simulink model "hcu_main_ADASwEPS"  (Simulink 8.2)
settings: Solver=FixedStepDiscrete  StartTime=0.0  StopTime=inf  FixedStep=0.001  RelTol=1e-3
PostLoadFcn:
  | , if any(exist('dsrtsu_mdlpostloadfcn', 'file') == [2, 3, 6]), try dsrtsu_mdlpostloadfcn('Execute', bdroot); catch fprintf('Error in PostLoadFcn (dsrtsu_mdlpostloadfcn) for model "%s":\n %s\n', bdroot, lasterr); end, end,
values from neighbouring files (symbols this model uses):
  C_TASK_1MS_S = (	C_TICK_TIME_S       )    [hcu_local_hdr.m]    (also in temp_ovrd_values.m = double(	0.001                  ))
  C_TASK_5MS_S = (	C_TICK_TIME_S      	)    [hcu_local_hdr.m]
  ENUM_ADASLFCSTATUS_OFF = uint8(  0  )    [hcu_local_hdr.m]
  ENUM_ADASLFCSTATUS_STANDBY = uint8(  1  )    [hcu_local_hdr.m]
  ENUM_ADASLKASTATUS_ACTIVE = uint8(  2  )    [hcu_local_hdr.m]
  ENUM_ADASLKASTATUS_OFF = uint8(  0  )    [hcu_local_hdr.m]
  ENUM_ADASLKASTATUS_STANDBY = uint8(  1  )    [hcu_local_hdr.m]
  ENUM_EPSMODEREQ_ANGLE = uint8(  1  )    [hcu_local_hdr.m]
  ENUM_EPSMODEREQ_INTERNAL = uint8(  0  )    [hcu_local_hdr.m]
  ENUM_EPSMODEREQ_TORQUE = uint8(  2  )    [hcu_local_hdr.m]
  ENUM_GEARPOSN_1ST = uint8(  1  )    [hcu_local_hdr.m]
  ENUM_GEARPOSN_2ND = uint8(  2  )    [hcu_local_hdr.m]
  ENUM_GEARPOSN_3RD = uint8(  3  )    [hcu_local_hdr.m]
  ENUM_GEARPOSN_4TH = uint8(  4  )    [hcu_local_hdr.m]
  ENUM_GEARPOSN_5TH = uint8(  5  )    [hcu_local_hdr.m]
  ENUM_GEARPOSN_6TH = uint8(  6  )    [hcu_local_hdr.m]
  ENUM_GEARPOSN_PN = uint8(  0  )    [hcu_local_hdr.m]
  ENUM_GEARPOSN_R = uint8(  7  )    [hcu_local_hdr.m]
  FALSE = boolean( 0 )    [hcu_local_hdr.m]
  TRUE = boolean( 1 )    [hcu_local_hdr.m]
undefined symbols (not defined in the file or in its folder): AACC_DistCtrlIMult_X_mps2, AACC_DistCtrlPMult_X_mps2, AACC_GearActual_enum, AACC_SpdCtrlIMult_X_mps2, AACC_SpdCtrlPMult_X_mps2, AACC_VehSpd_kph, AISP_EPSCurrent_pct, AISP_TqASensorDelta_pct, AISP_TqBSensorDelta_pct, ENUM_ACCSTATUS_ACTIVE, ENUM_ACCSTATUS_OFF, ENUM_ACCSTATUS_STANDBY, ENUM_ADASLFCSTATUS_ACTIVE, ENUM_ADASLFCSTATUS_TRANSITION, ENUM_LFCCCONTSTATUS_ACTIVE, ENUM_LFCCCONTSTATUS_NOTAVAIL_TEMP, ENUM_LFCCCONTSTATUS_OFF, ENUM_LFCCCONTSTATUS_READY, ENUM_LFCCCONTSTATUS_TRANSITION, ENUM_LKACCONTSTATUS_ACTIVE, ENUM_LKACCONTSTATUS_NOTAVAIL_TEMP, ENUM_LKACCONTSTATUS_OFF, ENUM_LKACCONTSTATUS_READY, KACC_AcclReqMax_g, KACC_AcclReqMin_g, KACC_ACCSetTimeGapDef1_s, KACC_ACCSetTimeGapDef2_s, KACC_ACCSetTimeGapDef3_s, KACC_ACCSetTimeGapDef4_s, KACC_ACCSetTimeGapDef5_s, KACC_AirDensity_kgpm3, KACC_AirDragCoef_rat, KACC_CommandsOn_flg, KACC_CruzSpdChgTimeThres_s, KACC_DecReqSwOffThres_Nm, KACC_DecReqSwOnThres_Nm, KACC_DistCtrlAdjTime_s, KACC_DistCtrlCalRate_s, KACC_DistCtrlIC_mps2, KACC_DistCtrlIGain_rat, KACC_DistCtrlIMax_mps2, KACC_DistCtrlIMin_mps2, KACC_DistCtrlIRest_flg, KACC_DistCtrlKGain_rat, KACC_DistCtrlPause_flg, KACC_DistCtrlPGain_rat, KACC_FinalDriveEff_pct, KACC_FinalDriveRatio_rat, KACC_FrontalArea_m2, KACC_GearBoxEff_pct, KACC_LongPushSpdChg_kph, KACC_MaxAccSetSpd_kph, KACC_MinAccSetSpd_kph, KACC_SetAllowSpdLim_kph, KACC_SpdCtrlAdjTime_s, KACC_SpdCtrlCalRate_s, KACC_SpdCtrlIC_mps2, KACC_SpdCtrlIGain_rat, KACC_SpdCtrlIMax_mps2, KACC_SpdCtrlIMin_mps2 ... (+26)
libraries: simulink x54, adas_lib x6, rti1401lib_dio_type3 x4, rtimmsu_dsrtlib x3, hcu_lib x2, aeb x1, ddm x1, dfr x1, dgi x1, dhp x1, dinr x1, dip x1
(part 4 of 9)

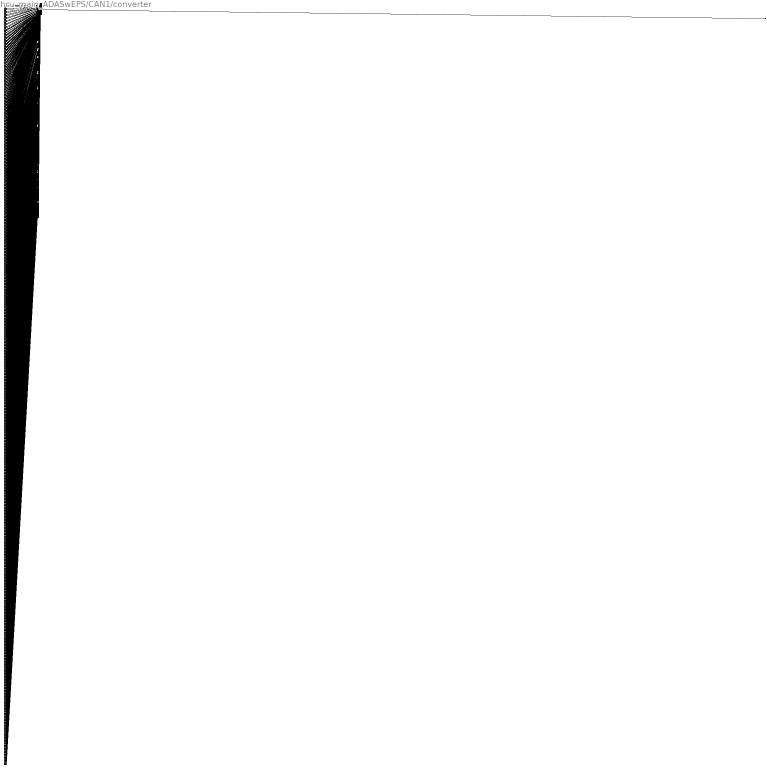
== system hcu_main_ADASwEPS/CAN1/converter ==
  in_1 : Inport
  in_2 : Inport  Port=2
  in_3 : Inport  Port=3
  in_4 : Inport  Port=4
  in_5 : Inport  Port=5
  in_6 : Inport  Port=6
  in_7 : Inport  Port=7
  in_8 : Inport  Port=8
  in_9 : Inport  Port=9
  in_10 : Inport  Port=10
  in_11 : Inport  Port=11
  in_12 : Inport  Port=12
  in_13 : Inport  Port=13
  in_14 : Inport  Port=14
  in_15 : Inport  Port=15
  in_16 : Inport  Port=16
  in_17 : Inport  Port=17
  in_18 : Inport  Port=18
  in_19 : Inport  Port=19
  in_20 : Inport  Port=20
  in_21 : Inport  Port=21
  in_22 : Inport  Port=22
  in_23 : Inport  Port=23
  in_24 : Inport  Port=24
  in_25 : Inport  Port=25
  in_26 : Inport  Port=26
  in_27 : Inport  Port=27
  in_28 : Inport  Port=28
  in_29 : Inport  Port=29
  in_30 : Inport  Port=30
  in_31 : Inport  Port=31
  in_32 : Inport  Port=32
  in_33 : Inport  Port=33
  in_34 : Inport  Port=34
  in_35 : Inport  Port=35
  in_36 : Inport  Port=36
  in_37 : Inport  Port=37
  in_38 : Inport  Port=38
  in_39 : Inport  Port=39
  in_40 : Inport  Port=40
  in_41 : Inport  Port=41
  in_42 : Inport  Port=42
  in_43 : Inport  Port=43
  in_44 : Inport  Port=44
  in_45 : Inport  Port=45
  in_46 : Inport  Port=46
  in_47 : Inport  Port=47
  in_48 : Inport  Port=48
  in_49 : Inport  Port=49
  in_50 : Inport  Port=50
  in_51 : Inport  Port=51
  in_52 : Inport  Port=52
  in_53 : Inport  Port=53
  in_54 : Inport  Port=54
  in_55 : Inport  Port=55
  in_56 : Inport  Port=56
  in_57 : Inport  Port=57
  in_58 : Inport  Port=58
  in_59 : Inport  Port=59
  in_60 : Inport  Port=60
  in_61 : Inport  Port=61
  in_62 : Inport  Port=62
  in_63 : Inport  Port=63
  in_64 : Inport  Port=64
  in_65 : Inport  Port=65
  in_66 : Inport  Port=66
  in_67 : Inport  Port=67
  in_68 : Inport  Port=68
  in_69 : Inport  Port=69
  in_70 : Inport  Port=70
  in_71 : Inport  Port=71
  in_72 : Inport  Port=72
  in_73 : Inport  Port=73
  in_74 : Inport  Port=74
  in_75 : Inport  Port=75
  in_76 : Inport  Port=76
  in_77 : Inport  Port=77
  in_78 : Inport  Port=78
  in_79 : Inport  Port=79
  in_80 : Inport  Port=80
  in_81 : Inport  Port=81
  in_82 : Inport  Port=82
  in_83 : Inport  Port=83
  in_84 : Inport  Port=84
  in_85 : Inport  Port=85
  in_86 : Inport  Port=86
  in_87 : Inport  Port=87
  in_88 : Inport  Port=88
  in_89 : Inport  Port=89
  in_90 : Inport  Port=90
  in_91 : Inport  Port=91
  in_92 : Inport  Port=92
  in_93 : Inport  Port=93
  in_94 : Inport  Port=94
  in_95 : Inport  Port=95
  in_96 : Inport  Port=96
  in_97 : Inport  Port=97
  in_98 : Inport  Port=98
  in_99 : Inport  Port=99
  in_100 : Inport  Port=100
  in_101 : Inport  Port=101
  in_102 : Inport  Port=102
  in_103 : Inport  Port=103
  in_104 : Inport  Port=104
  in_105 : Inport  Port=105
  in_106 : Inport  Port=106
  in_107 : Inport  Port=107
  in_108 : Inport  Port=108
  in_109 : Inport  Port=109
  in_110 : Inport  Port=110
  in_111 : Inport  Port=111
  in_112 : Inport  Port=112
  in_113 : Inport  Port=113
  in_114 : Inport  Port=114
  in_115 : Inport  Port=115
  in_116 : Inport  Port=116
  in_117 : Inport  Port=117
  in_118 : Inport  Port=118
  in_119 : Inport  Port=119
  in_120 : Inport  Port=120
  in_121 : Inport  Port=121
  in_122 : Inport  Port=122
  in_123 : Inport  Port=123
  in_124 : Inport  Port=124
  in_125 : Inport  Port=125
  in_126 : Inport  Port=126
  in_127 : Inport  Port=127
  in_128 : Inport  Port=128
  in_129 : Inport  Port=129
  in_130 : Inport  Port=130
  in_131 : Inport  Port=131
  in_132 : Inport  Port=132
  in_133 : Inport  Port=133
  in_134 : Inport  Port=134
  in_135 : Inport  Port=135
  in_136 : Inport  Port=136
  in_137 : Inport  Port=137
  in_138 : Inport  Port=138
  in_139 : Inport  Port=139
  in_140 : Inport  Port=140
  in_141 : Inport  Port=141
  in_142 : Inport  Port=142
  in_143 : Inport  Port=143
  in_144 : Inport  Port=144
  in_145 : Inport  Port=145
  in_146 : Inport  Port=146
  in_147 : Inport  Port=147
  in_148 : Inport  Port=148
  in_149 : Inport  Port=149
  in_150 : Inport  Port=150
  in_151 : Inport  Port=151
  in_152 : Inport  Port=152
  in_153 : Inport  Port=153
  in_154 : Inport  Port=154
  in_155 : Inport  Port=155
  in_156 : Inport  Port=156
  in_157 : Inport  Port=157
  in_158 : Inport  Port=158
  in_159 : Inport  Port=159
  in_160 : Inport  Port=160
  in_161 : Inport  Port=161
  in_162 : Inport  Port=162
  in_163 : Inport  Port=163
  in_164 : Inport  Port=164
  in_165 : Inport  Port=165
  in_166 : Inport  Port=166
  in_167 : Inport  Port=167
  in_168 : Inport  Port=168
  in_169 : Inport  Port=169
  in_170 : Inport  Port=170
  in_171 : Inport  Port=171
  in_172 : Inport  Port=172
  in_173 : Inport  Port=173
  in_174 : Inport  Port=174
  in_175 : Inport  Port=175
  in_176 : Inport  Port=176
  in_177 : Inport  Port=177
  in_178 : Inport  Port=178
  in_179 : Inport  Port=179
  in_180 : Inport  Port=180
  in_181 : Inport  Port=181
  in_182 : Inport  Port=182
  in_183 : Inport  Port=183
  in_184 : Inport  Port=184
  in_185 : Inport  Port=185
  in_186 : Inport  Port=186
  in_187 : Inport  Port=187
  in_188 : Inport  Port=188
  in_189 : Inport  Port=189
  in_190 : Inport  Port=190
  in_191 : Inport  Port=191
  in_192 : Inport  Port=192
  in_193 : Inport  Port=193
  in_194 : Inport  Port=194
  in_195 : Inport  Port=195
  in_196 : Inport  Port=196
  in_197 : Inport  Port=197
  in_198 : Inport  Port=198
  in_199 : Inport  Port=199
  in_200 : Inport  Port=200
  in_201 : Inport  Port=201
  in_202 : Inport  Port=202
  in_203 : Inport  Port=203
  in_204 : Inport  Port=204
  in_205 : Inport  Port=205
  in_206 : Inport  Port=206
  in_207 : Inport  Port=207
  in_208 : Inport  Port=208
  in_209 : Inport  Port=209
  in_210 : Inport  Port=210
  in_211 : Inport  Port=211
  in_212 : Inport  Port=212
  in_213 : Inport  Port=213
  in_214 : Inport  Port=214
  in_215 : Inport  Port=215
  in_216 : Inport  Port=216
  in_217 : Inport  Port=217
  in_218 : Inport  Port=218
  in_219 : Inport  Port=219
  in_220 : Inport  Port=220
  in_221 : Inport  Port=221
  in_222 : Inport  Port=222
  in_223 : Inport  Port=223
  in_224 : Inport  Port=224
  in_225 : Inport  Port=225
  in_226 : Inport  Port=226
  in_227 : Inport  Port=227
  in_228 : Inport  Port=228
  in_229 : Inport  Port=229
  in_230 : Inport  Port=230
  in_231 : Inport  Port=231
  in_232 : Inport  Port=232
  in_233 : Inport  Port=233
  in_234 : Inport  Port=234
  in_235 : Inport  Port=235
  in_236 : Inport  Port=236
  in_237 : Inport  Port=237
  in_238 : Inport  Port=238
  in_239 : Inport  Port=239
  in_240 : Inport  Port=240
  in_241 : Inport  Port=241
  in_242 : Inport  Port=242
  in_243 : Inport  Port=243
  in_244 : Inport  Port=244
  in_245 : Inport  Port=245
  in_246 : Inport  Port=246
  in_247 : Inport  Port=247
  in_248 : Inport  Port=248
  in_249 : Inport  Port=249
  in_250 : Inport  Port=250
  in_251 : Inport  Port=251
  in_252 : Inport  Port=252
  in_253 : Inport  Port=253
  in_254 : Inport  Port=254
  in_255 : Inport  Port=255
  in_256 : Inport  Port=256
  in_257 : Inport  Port=257
  in_258 : Inport  Port=258
  in_259 : Inport  Port=259
  in_260 : Inport  Port=260
  in_261 : Inport  Port=261
  in_262 : Inport  Port=262
  in_263 : Inport  Port=263
  in_264 : Inport  Port=264
  in_265 : Inport  Port=265
  in_266 : Inport  Port=266
  in_267 : Inport  Port=267
  in_268 : Inport  Port=268
  in_269 : Inport  Port=269
  in_270 : Inport  Port=270
  in_271 : Inport  Port=271
  in_272 : Inport  Port=272
  in_273 : Inport  Port=273
  in_274 : Inport  Port=274
  in_275 : Inport  Port=275
  in_276 : Inport  Port=276
  in_277 : Inport  Port=277
  in_278 : Inport  Port=278
  in_279 : Inport  Port=279
  in_280 : Inport  Port=280
  in_281 : Inport  Port=281
  in_282 : Inport  Port=282
  in_283 : Inport  Port=283
  in_284 : Inport  Port=284
  in_285 : Inport  Port=285
  in_286 : Inport  Port=286
  in_287 : Inport  Port=287
  in_288 : Inport  Port=288
  in_289 : Inport  Port=289
  in_290 : Inport  Port=290
  in_291 : Inport  Port=291
  in_292 : Inport  Port=292
  in_293 : Inport  Port=293
  in_294 : Inport  Port=294
  in_295 : Inport  Port=295
  in_296 : Inport  Port=296
  in_297 : Inport  Port=297
  in_298 : Inport  Port=298
  in_299 : Inport  Port=299
  in_300 : Inport  Port=300
  in_301 : Inport  Port=301
  in_302 : Inport  Port=302
  in_303 : Inport  Port=303
  in_304 : Inport  Port=304
  in_305 : Inport  Port=305
  in_306 : Inport  Port=306
  in_307 : Inport  Port=307
  in_308 : Inport  Port=308
  in_309 : Inport  Port=309
  in_310 : Inport  Port=310
  in_311 : Inport  Port=311
  in_312 : Inport  Port=312
  in_313 : Inport  Port=313
  in_314 : Inport  Port=314
  in_315 : Inport  Port=315
  in_316 : Inport  Port=316
  in_317 : Inport  Port=317
  in_318 : Inport  Port=318
  in_319 : Inport  Port=319
  in_320 : Inport  Port=320
  in_321 : Inport  Port=321
  in_322 : Inport  Port=322
  in_323 : Inport  Port=323
  in_324 : Inport  Port=324
  in_325 : Inport  Port=325
  in_326 : Inport  Port=326
  in_327 : Inport  Port=327
  in_328 : Inport  Port=328
  in_329 : Inport  Port=329
  in_330 : Inport  Port=330
  in_331 : Inport  Port=331
  in_332 : Inport  Port=332
  in_333 : Inport  Port=333
  in_334 : Inport  Port=334
  in_335 : Inport  Port=335
  in_336 : Inport  Port=336
  in_337 : Inport  Port=337
  in_338 : Inport  Port=338
  in_339 : Inport  Port=339
  in_340 : Inport  Port=340
  in_341 : Inport  Port=341
  in_342 : Inport  Port=342
  in_343 : Inport  Port=343
  in_344 : Inport  Port=344
  in_345 : Inport  Port=345
  in_346 : Inport  Port=346
  in_347 : Inport  Port=347
  in_348 : Inport  Port=348
  in_349 : Inport  Port=349
  in_350 : Inport  Port=350
  in_351 : Inport  Port=351
  in_352 : Inport  Port=352
  in_353 : Inport  Port=353
  in_354 : Inport  Port=354
  in_355 : Inport  Port=355
  in_356 : Inport  Port=356
  in_357 : Inport  Port=357
  in_358 : Inport  Port=358
  in_359 : Inport  Port=359
  in_360 : Inport  Port=360
  in_361 : Inport  Port=361
  in_362 : Inport  Port=362
  in_363 : Inport  Port=363
  in_364 : Inport  Port=364
  in_365 : Inport  Port=365
  in_366 : Inport  Port=366
  in_367 : Inport  Port=367
  in_368 : Inport  Port=368
  in_369 : Inport  Port=369
  in_370 : Inport  Port=370
  in_371 : Inport  Port=371
  in_372 : Inport  Port=372
  in_373 : Inport  Port=373
  in_374 : Inport  Port=374
  in_375 : Inport  Port=375
  in_376 : Inport  Port=376
  in_377 : Inport  Port=377
  in_378 : Inport  Port=378
  in_379 : Inport  Port=379
  in_380 : Inport  Port=380
  in_381 : Inport  Port=381
  in_382 : Inport  Port=382
  in_383 : Inport  Port=383
  in_384 : Inport  Port=384
  in_385 : Inport  Port=385
  in_386 : Inport  Port=386
  in_387 : Inport  Port=387
  in_388 : Inport  Port=388
  in_389 : Inport  Port=389
  in_390 : Inport  Port=390
  in_391 : Inport  Port=391
  in_392 : Inport  Port=392
  in_393 : Inport  Port=393
  in_394 : Inport  Port=394
  in_395 : Inport  Port=395
  in_396 : Inport  Port=396
  in_397 : Inport  Port=397
  in_398 : Inport  Port=398
  in_399 : Inport  Port=399
  in_400 : Inport  Port=400
  in_401 : Inport  Port=401
  in_402 : Inport  Port=402
  in_403 : Inport  Port=403
  in_404 : Inport  Port=404
  in_405 : Inport  Port=405
  in_406 : Inport  Port=406
  in_407 : Inport  Port=407
  in_408 : Inport  Port=408
  in_409 : Inport  Port=409
  in_410 : Inport  Port=410
  in_411 : Inport  Port=411
  in_412 : Inport  Port=412
  in_413 : Inport  Port=413
  in_414 : Inport  Port=414
  in_415 : Inport  Port=415
  in_416 : Inport  Port=416
  in_417 : Inport  Port=417
  in_418 : Inport  Port=418
  in_419 : Inport  Port=419
  in_420 : Inport  Port=420
  in_421 : Inport  Port=421
  in_422 : Inport  Port=422
  in_423 : Inport  Port=423
  in_424 : Inport  Port=424
  in_425 : Inport  Port=425
  in_426 : Inport  Port=426
  in_427 : Inport  Port=427
  in_428 : Inport  Port=428
  in_429 : Inport  Port=429
  in_430 : Inport  Port=430
  in_431 : Inport  Port=431
  in_432 : Inport  Port=432
  in_433 : Inport  Port=433
  in_434 : Inport  Port=434
  in_435 : Inport  Port=435
  in_436 : Inport  Port=436
  in_437 : Inport  Port=437
  in_438 : Inport  Port=438
  in_439 : Inport  Port=439
  in_440 : Inport  Port=440
  in_441 : Inport  Port=441
  in_442 : Inport  Port=442
  in_443 : Inport  Port=443
  in_444 : Inport  Port=444
  in_445 : Inport  Port=445
  in_446 : Inport  Port=446
  in_447 : Inport  Port=447
  in_448 : Inport  Port=448
  in_449 : Inport  Port=449
  in_450 : Inport  Port=450
  in_451 : Inport  Port=451
  in_452 : Inport  Port=452
  in_453 : Inport  Port=453
  in_454 : Inport  Port=454
  in_455 : Inport  Port=455
  in_456 : Inport  Port=456
  in_457 : Inport  Port=457
  in_458 : Inport  Port=458
  in_459 : Inport  Port=459
  in_460 : Inport  Port=460
  in_461 : Inport  Port=461
  in_462 : Inport  Port=462
  in_463 : Inport  Port=463
  in_464 : Inport  Port=464
  in_465 : Inport  Port=465
  in_466 : Inport  Port=466
  in_467 : Inport  Port=467
  in_468 : Inport  Port=468
  in_469 : Inport  Port=469
  in_470 : Inport  Port=470
  in_471 : Inport  Port=471
  in_472 : Inport  Port=472
  in_473 : Inport  Port=473
  in_474 : Inport  Port=474
  in_475 : Inport  Port=475
  in_476 : Inport  Port=476
  in_477 : Inport  Port=477
  in_478 : Inport  Port=478
  in_479 : Inport  Port=479
  in_480 : Inport  Port=480
  in_481 : Inport  Port=481
  in_482 : Inport  Port=482
  in_483 : Inport  Port=483
  in_484 : Inport  Port=484
  in_485 : Inport  Port=485
  in_486 : Inport  Port=486
  in_487 : Inport  Port=487
  in_488 : Inport  Port=488
  in_489 : Inport  Port=489
  in_490 : Inport  Port=490
  in_491 : Inport  Port=491
  in_492 : Inport  Port=492
  in_493 : Inport  Port=493
  in_494 : Inport  Port=494
  in_495 : Inport  Port=495
  in_496 : Inport  Port=496
  in_497 : Inport  Port=497
  in_498 : Inport  Port=498
  in_499 : Inport  Port=499
  in_500 : Inport  Port=500
  in_501 : Inport  Port=501
  in_502 : Inport  Port=502
  in_503 : Inport  Port=503
  in_504 : Inport  Port=504
  in_505 : Inport  Port=505
  in_506 : Inport  Port=506
  in_507 : Inport  Port=507
  in_508 : Inport  Port=508
  in_509 : Inport  Port=509
  in_510 : Inport  Port=510
  in_511 : Inport  Port=511
  in_512 : Inport  Port=512
  in_513 : Inport  Port=513
  in_514 : Inport  Port=514
  ABS1 : BusCreator  Inputs=22
  ABS2 : BusCreator  Inputs=26
  ABS3 : BusCreator  Inputs=19
  ABS4 : BusCreator  Inputs=21
  AC1 : BusCreator  Inputs=12
  ADAS1 : BusCreator  Inputs=12
  ADAS3 : BusCreator  Inputs=13
  BCM1 : BusCreator  Inputs=21
  BCM2 : BusCreator  Inputs=12
  ECM1 : BusCreator  Inputs=18
  ECM2 : BusCreator  Inputs=13
  ECM3 : BusCreator  Inputs=19
  ECM9 : BusCreator  Inputs=16
  EPAS2 : BusCreator  Inputs=19
  EPAS3 : BusCreator  Inputs=26
  EPB1 : BusCreator  Inputs=12
  HCU3 : BusCreator  Inputs=27
  HCU4 : BusCreator  Inputs=21
  HMI1 : BusCreator  Inputs=33
  HMI2 : BusCreator  Inputs=18
  Meter1 : BusCreator  Inputs=15
  Meter3 : BusCreator  Inputs=12
  Mux : BusCreator  Inputs=28
  NMmADAS : BusCreator  Inputs=15
  SAS1 : BusCreator  Inputs=16
  TCM1 : BusCreator  Inputs=19
  TCM2 : BusCreator  Inputs=12
  VCU1 : BusCreator  Inputs=28
  VCU2 : BusCreator  Inputs=17
  out : Outport
  wires:
  in_1/1 -> ABS1/1  "BoosterVac"
  ABS1/1 -> Mux/1  "ABS1"
  in_2/1 -> ABS1/2  "GRADE"
  in_3/1 -> ABS1/3  "BoosterVac_Failed"
  in_4/1 -> ABS1/4  "BoosterVac_Sta"
  in_5/1 -> ABS1/5  "BoosterVac_V"
  in_6/1 -> ABS1/6  "GRADE_V"
  in_7/1 -> ABS1/7  "TCSReqVal_V"
  in_8/1 -> ABS1/8  "TCSReqStrat"
  in_9/1 -> ABS1/9  "TCSRollCnt"
  in_10/1 -> ABS1/10  "TCSReqProt"
  in_11/1 -> ABS1/11  "TCSReqVal"
  in_12/1 -> ABS1/12  "RX_Status"
  in_13/1 -> ABS1/13  "RX_Time"
  in_14/1 -> ABS1/14  "RX_DeltaTime"
  in_15/1 -> ABS1/15  "RAW_Byte_1"
  in_16/1 -> ABS1/16  "RAW_Byte_2"
  in_17/1 -> ABS1/17  "RAW_Byte_3"
  in_18/1 -> ABS1/18  "RAW_Byte_4"
  in_19/1 -> ABS1/19  "RAW_Byte_5"
  in_20/1 -> ABS1/20  "RAW_Byte_6"
  in_21/1 -> ABS1/21  "RAW_Byte_7"
  in_22/1 -> ABS1/22  "RAW_Byte_8"
  in_23/1 -> ABS2/1  "VehSpeed_Checksum"
  ABS2/1 -> Mux/2  "ABS2"
  in_24/1 -> ABS2/2  "VehSpeed_LifeCount"
  in_25/1 -> ABS2/3  "HSA_Failed"
  in_26/1 -> ABS2/4  "HSA_Active"
  in_27/1 -> ABS2/5  "BrkSw_Sta"
  in_28/1 -> ABS2/6  "BrkSw_V"
  in_29/1 -> ABS2/7  "EBD_Failed"
  in_30/1 -> ABS2/8  "TCS_Enabled"
  in_31/1 -> ABS2/9  "TCS_Failed"
  in_32/1 -> ABS2/10  "ESC_Failed"
  in_33/1 -> ABS2/11  "ABS_Failed"
  in_34/1 -> ABS2/12  "TCS_Active"
  in_35/1 -> ABS2/13  "ESC_Active"
  in_36/1 -> ABS2/14  "ABS_Active"
  in_37/1 -> ABS2/15  "VehSpeed"
  in_38/1 -> ABS2/16  "RX_Status"
  in_39/1 -> ABS2/17  "RX_Time"
  in_40/1 -> ABS2/18  "RX_DeltaTime"
  in_41/1 -> ABS2/19  "RAW_Byte_1"
  in_42/1 -> ABS2/20  "RAW_Byte_2"
  in_43/1 -> ABS2/21  "RAW_Byte_3"
  in_44/1 -> ABS2/22  "RAW_Byte_4"
  in_45/1 -> ABS2/23  "RAW_Byte_5"
  in_46/1 -> ABS2/24  "RAW_Byte_6"
  in_47/1 -> ABS2/25  "RAW_Byte_7"
  in_48/1 -> ABS2/26  "RAW_Byte_8"
  in_49/1 -> ABS3/1  "LF_RawWhlSpeed_V"
  ABS3/1 -> Mux/3  "ABS3"
  in_50/1 -> ABS3/2  "LF_RawWhlSpeed"
  in_51/1 -> ABS3/3  "RF_RawWhlSpeed_V"
  in_52/1 -> ABS3/4  "RF_RawWhlSpeed"
  in_53/1 -> ABS3/5  "LR_RawWhlSpeed_V"
  in_54/1 -> ABS3/6  "LR_RawWhlSpeed"
  in_55/1 -> ABS3/7  "RR_RawWhlSpeed_V"
  in_56/1 -> ABS3/8  "RR_RawWhlSpeed"
  in_57/1 -> ABS3/9  "RX_Status"
  in_58/1 -> ABS3/10  "RX_Time"
  in_59/1 -> ABS3/11  "RX_DeltaTime"
  in_60/1 -> ABS3/12  "RAW_Byte_1"
  in_61/1 -> ABS3/13  "RAW_Byte_2"
  in_62/1 -> ABS3/14  "RAW_Byte_3"
  in_63/1 -> ABS3/15  "RAW_Byte_4"
  in_64/1 -> ABS3/16  "RAW_Byte_5"
  in_65/1 -> ABS3/17  "RAW_Byte_6"
  in_66/1 -> ABS3/18  "RAW_Byte_7"
  in_67/1 -> ABS3/19  "RAW_Byte_8"
  in_68/1 -> ABS4/1  "LongAccel"
  ABS4/1 -> Mux/4  "ABS4"
  in_69/1 -> ABS4/2  "SteerAng"
  in_70/1 -> ABS4/3  "YawRate"
  in_71/1 -> ABS4/4  "LatAccel"
  in_72/1 -> ABS4/5  "MCPressure"
  in_73/1 -> ABS4/6  "MCPressure_V"
  in_74/1 -> ABS4/7  "LongAccel_V"
  in_75/1 -> ABS4/8  "LatAccel_V"
  in_76/1 -> ABS4/9  "YawRate_V"
  in_77/1 -> ABS4/10  "SteerAng_V"
  in_78/1 -> ABS4/11  "RX_Status"
  in_79/1 -> ABS4/12  "RX_Time"
  in_80/1 -> ABS4/13  "RX_DeltaTime"
  in_81/1 -> ABS4/14  "RAW_Byte_1"
  in_82/1 -> ABS4/15  "RAW_Byte_2"
  in_83/1 -> ABS4/16  "RAW_Byte_3"
  in_84/1 -> ABS4/17  "RAW_Byte_4"
  in_85/1 -> ABS4/18  "RAW_Byte_5"
  in_86/1 -> ABS4/19  "RAW_Byte_6"
  in_87/1 -> ABS4/20  "RAW_Byte_7"
  in_88/1 -> ABS4/21  "RAW_Byte_8"
  in_89/1 -> AC1/1  "Sta_Out_Temp"
  AC1/1 -> Mux/5  "AC1"
  in_90/1 -> AC1/2  "RX_Status"
  in_91/1 -> AC1/3  "RX_Time"
  in_92/1 -> AC1/4  "RX_DeltaTime"
  in_93/1 -> AC1/5  "RAW_Byte_1"
  in_94/1 -> AC1/6  "RAW_Byte_2"
  in_95/1 -> AC1/7  "RAW_Byte_3"
  in_96/1 -> AC1/8  "RAW_Byte_4"
  in_97/1 -> AC1/9  "RAW_Byte_5"
  in_98/1 -> AC1/10  "RAW_Byte_6"
  in_99/1 -> AC1/11  "RAW_Byte_7"
  in_100/1 -> AC1/12  "RAW_Byte_8"
  in_101/1 -> ADAS1/1  "ADAS1_Checksum"
  ADAS1/1 -> Mux/6  "ADAS1"
  in_102/1 -> ADAS1/2  "ADAS1_LifeCount"
  in_103/1 -> ADAS1/3  "ADAS_StrTqReq_A"
  in_104/1 -> ADAS1/4  "ADAS_StrAngReq_A"
  in_105/1 -> ADAS1/5  "ADAS_LFCTransGain_A"
  in_106/1 -> ADAS1/6  "ADAS_EPSMode"
  in_107/1 -> ADAS1/7  "ADAS_LKAStatus"
  in_108/1 -> ADAS1/8  "ADAS_LFCMode"
  in_109/1 -> ADAS1/9  "ADAS_LFCStatus"
  in_110/1 -> ADAS1/10  "ADAS_StrTqReq"
  in_111/1 -> ADAS1/11  "ADAS_LFCTransGain"
  in_112/1 -> ADAS1/12  "ADAS_StrAngReq"
  in_113/1 -> ADAS3/1  "ADAS3_Checksum"
  ADAS3/1 -> Mux/7  "ADAS3"
  in_114/1 -> ADAS3/2  "ADAS3_LifeCount"
  in_115/1 -> ADAS3/3  "ForceLowBeam"
  in_116/1 -> ADAS3/4  "LeftTurnLightReq"
  in_117/1 -> ADAS3/5  "RightTurnLightReq"
  in_118/1 -> ADAS3/6  "HazardWarningReq"
  in_119/1 -> ADAS3/7  "ADAS_MIL"
  in_120/1 -> ADAS3/8  "ADAS_ShftPosnReq_A"
  in_121/1 -> ADAS3/9  "ADAS_ShftPosnReq"
  in_122/1 -> ADAS3/10  "ADAS_VehSpdLim_A"
  in_123/1 -> ADAS3/11  "ADAS_GearPosnReq_A"
  in_124/1 -> ADAS3/12  "ADAS_GearPosnReq"
  in_125/1 -> ADAS3/13  "ADAS_VehSpdLim"
  in_126/1 -> BCM1/1  "BCM_Hazard_Sta"
  BCM1/1 -> Mux/8  "BCM1"
  in_127/1 -> BCM1/2  "BCM_LRDrSw_Sta"
  in_128/1 -> BCM1/3  "BCM_RRDrSw_Sta"
  in_129/1 -> BCM1/4  "BCM_TGateSw_Sta"
  in_130/1 -> BCM1/5  "BCM_RTurnLp_Sta"
  in_131/1 -> BCM1/6  "BCM_LTurnLp_Sta"
  in_132/1 -> BCM1/7  "BCM_AllDrSw_Sta"
  in_133/1 -> BCM1/8  "BCM_PDrSw_Sta"
  in_134/1 -> BCM1/9  "BCM_DDrSw_Sta"
  in_135/1 -> BCM1/10  "BCM_Key_Sta"
  in_136/1 -> BCM1/11  "RX_Status"
  in_137/1 -> BCM1/12  "RX_Time"
  in_138/1 -> BCM1/13  "RX_DeltaTime"
  in_139/1 -> BCM1/14  "RAW_Byte_1"
  in_140/1 -> BCM1/15  "RAW_Byte_2"
  in_141/1 -> BCM1/16  "RAW_Byte_3"
  in_142/1 -> BCM1/17  "RAW_Byte_4"
  in_143/1 -> BCM1/18  "RAW_Byte_5"
  in_144/1 -> BCM1/19  "RAW_Byte_6"
  in_145/1 -> BCM1/20  "RAW_Byte_7"
  in_146/1 -> BCM1/21  "RAW_Byte_8"
  in_147/1 -> BCM2/1  "BCM_SRS_Crash_Info"
  BCM2/1 -> Mux/9  "BCM2"
  in_148/1 -> BCM2/2  "RX_Status"
  in_149/1 -> BCM2/3  "RX_Time"
  in_150/1 -> BCM2/4  "RX_DeltaTime"
  in_151/1 -> BCM2/5  "RAW_Byte_1"
  in_152/1 -> BCM2/6  "RAW_Byte_2"
  in_153/1 -> BCM2/7  "RAW_Byte_3"
  in_154/1 -> BCM2/8  "RAW_Byte_4"
  in_155/1 -> BCM2/9  "RAW_Byte_5"
  in_156/1 -> BCM2/10  "RAW_Byte_6"
  in_157/1 -> BCM2/11  "RAW_Byte_7"
  in_158/1 -> BCM2/12  "RAW_Byte_8"
  in_159/1 -> ECM1/1  "CAN_TQ_STND"
  ECM1/1 -> Mux/10  "ECM1"
  in_160/1 -> ECM1/2  "CAN_TQFR"
  in_161/1 -> ECM1/3  "CAN_TQI"
  in_162/1 -> ECM1/4  "CAN_N"
  in_163/1 -> ECM1/5  "CAN_TQI_ACOR"
  in_164/1 -> ECM1/6  "LV_CAN_N_ERR"
  in_165/1 -> ECM1/7  "LV_CAN_SUB_TQI"
  in_166/1 -> ECM1/8  "RX_Status"
  in_167/1 -> ECM1/9  "RX_Time"
  in_168/1 -> ECM1/10  "RX_DeltaTime"
  in_169/1 -> ECM1/11  "RAW_Byte_1"
  in_170/1 -> ECM1/12  "RAW_Byte_2"
  in_171/1 -> ECM1/13  "RAW_Byte_3"
  in_172/1 -> ECM1/14  "RAW_Byte_4"
  in_173/1 -> ECM1/15  "RAW_Byte_5"
  in_174/1 -> ECM1/16  "RAW_Byte_6"
  in_175/1 -> ECM1/17  "RAW_Byte_7"
  in_176/1 -> ECM1/18  "RAW_Byte_8"
  in_177/1 -> ECM2/1  "Eng_Hood_SW"
  ECM2/1 -> Mux/11  "ECM2"
  in_178/1 -> ECM2/2  "LV_CAN_ENG_RUN_ST"
  in_179/1 -> ECM2/3  "RX_Status"
  in_180/1 -> ECM2/4  "RX_Time"
  in_181/1 -> ECM2/5  "RX_DeltaTime"
  in_182/1 -> ECM2/6  "RAW_Byte_1"
  in_183/1 -> ECM2/7  "RAW_Byte_2"
  in_184/1 -> ECM2/8  "RAW_Byte_3"
  in_185/1 -> ECM2/9  "RAW_Byte_4"
  in_186/1 -> ECM2/10  "RAW_Byte_5"
  in_187/1 -> ECM2/11  "RAW_Byte_6"
  in_188/1 -> ECM2/12  "RAW_Byte_7"
  in_189/1 -> ECM2/13  "RAW_Byte_8"
  in_190/1 -> ECM3/1  "CAN_PV_AV"
  ECM3/1 -> Mux/12  "ECM3"
  in_191/1 -> ECM3/2  "CAN_PV_EFC"
  in_192/1 -> ECM3/3  "LV_CAN_MAIN_CRU_ER"
  in_193/1 -> ECM3/4  "LV_CAN_MAIN_CRU"
  in_194/1 -> ECM3/5  "LV_CAN_SET_CRU_ERR"
  in_195/1 -> ECM3/6  "LV_CAN_SET_CRU"
  in_196/1 -> ECM3/7  "LV_CAN_ERRPAS"
  in_197/1 -> ECM3/8  "LV_CAN_ERRPVS"
  in_198/1 -> ECM3/9  "RX_Status"
  in_199/1 -> ECM3/10  "RX_Time"
  in_200/1 -> ECM3/11  "RX_DeltaTime"
  in_201/1 -> ECM3/12  "RAW_Byte_1"
  in_202/1 -> ECM3/13  "RAW_Byte_2"
  in_203/1 -> ECM3/14  "RAW_Byte_3"
  in_204/1 -> ECM3/15  "RAW_Byte_4"
  in_205/1 -> ECM3/16  "RAW_Byte_5"
  in_206/1 -> ECM3/17  "RAW_Byte_6"
  in_207/1 -> ECM3/18  "RAW_Byte_7"
  in_208/1 -> ECM3/19  "RAW_Byte_8"
  in_209/1 -> ECM9/1  "EngTqMin"
  ECM9/1 -> Mux/13  "ECM9"
  in_210/1 -> ECM9/2  "EngTqMax"
  in_211/1 -> ECM9/3  "EMSOpState"
  in_212/1 -> ECM9/4  "EMSHybridOpState"
  in_213/1 -> ECM9/5  "ECM9RollCnt"
  in_214/1 -> ECM9/6  "RX_Status"
  in_215/1 -> ECM9/7  "RX_Time"
  in_216/1 -> ECM9/8  "RX_DeltaTime"
  in_217/1 -> ECM9/9  "RAW_Byte_1"
  in_218/1 -> ECM9/10  "RAW_Byte_2"
  in_219/1 -> ECM9/11  "RAW_Byte_3"
  in_220/1 -> ECM9/12  "RAW_Byte_4"
  in_221/1 -> ECM9/13  "RAW_Byte_5"
  in_222/1 -> ECM9/14  "RAW_Byte_6"
  in_223/1 -> ECM9/15  "RAW_Byte_7"
  in_224/1 -> ECM9/16  "RAW_Byte_8"
  in_225/1 -> EPAS2/1  "SAS_CheckSum2"
  EPAS2/1 -> Mux/14  "EPAS2"
  in_226/1 -> EPAS2/2  "SAS_MsgCount2"
  in_227/1 -> EPAS2/3  "R_SAS_Angle"
  in_228/1 -> EPAS2/4  "Steering_Torque"
  in_229/1 -> EPAS2/5  "Steering_Torque_V"
  in_230/1 -> EPAS2/6  "RSP_OK"
  in_231/1 -> EPAS2/7  "EpasFailed"
  in_232/1 -> EPAS2/8  "Elect_PWR_Consumpt"
  in_233/1 -> EPAS2/9  "RX_Status"
  in_234/1 -> EPAS2/10  "RX_Time"
  in_235/1 -> EPAS2/11  "RX_DeltaTime"
  in_236/1 -> EPAS2/12  "RAW_Byte_1"
  in_237/1 -> EPAS2/13  "RAW_Byte_2"
  in_238/1 -> EPAS2/14  "RAW_Byte_3"
  in_239/1 -> EPAS2/15  "RAW_Byte_4"
  in_240/1 -> EPAS2/16  "RAW_Byte_5"
  in_241/1 -> EPAS2/17  "RAW_Byte_6"
  in_242/1 -> EPAS2/18  "RAW_Byte_7"
  in_243/1 -> EPAS2/19  "RAW_Byte_8"
  in_244/1 -> EPAS3/1  "EPAS3_Checksum"
  EPAS3/1 -> Mux/15  "EPAS3"
  in_245/1 -> EPAS3/2  "EPAS3_LifeCount"
  in_246/1 -> EPAS3/3  "EPSLFCFailed"
  in_247/1 -> EPAS3/4  "CurStrTqReq_A"
  in_248/1 -> EPAS3/5  "CurStrAngReq_A"
  in_249/1 -> EPAS3/6  "EPSLFCStatus"
  in_250/1 -> EPAS3/7  "EPSBattVolt"
  in_251/1 -> EPAS3/8  "CurStrTqReq"
  in_252/1 -> EPAS3/9  "DriverStrIntdLvl"
  in_253/1 -> EPAS3/10  "DriverStrIntd"
  in_254/1 -> EPAS3/11  "EPSLFCAbReason"
  in_255/1 -> EPAS3/12  "EPSLKAAbReason"
  in_256/1 -> EPAS3/13  "EPSLKAFailed"
  in_257/1 -> EPAS3/14  "EPSLKAStatus"
  in_258/1 -> EPAS3/15  "CurStrAngReq"
  in_259/1 -> EPAS3/16  "RX_Status"
  in_260/1 -> EPAS3/17  "RX_Time"
  in_261/1 -> EPAS3/18  "RX_DeltaTime"
  in_262/1 -> EPAS3/19  "RAW_Byte_1"
  in_263/1 -> EPAS3/20  "RAW_Byte_2"
  in_264/1 -> EPAS3/21  "RAW_Byte_3"
  in_265/1 -> EPAS3/22  "RAW_Byte_4"
  in_266/1 -> EPAS3/23  "RAW_Byte_5"
  in_267/1 -> EPAS3/24  "RAW_Byte_6"
  in_268/1 -> EPAS3/25  "RAW_Byte_7"
  in_269/1 -> EPAS3/26  "RAW_Byte_8"
  in_270/1 -> EPB1/1  "PB_BrakeBinStat"
  EPB1/1 -> Mux/16  "EPB1"
  in_271/1 -> EPB1/2  "RX_Status"
  in_272/1 -> EPB1/3  "RX_Time"
  in_273/1 -> EPB1/4  "RX_DeltaTime"
  in_274/1 -> EPB1/5  "RAW_Byte_1"
  in_275/1 -> EPB1/6  "RAW_Byte_2"
  in_276/1 -> EPB1/7  "RAW_Byte_3"
  in_277/1 -> EPB1/8  "RAW_Byte_4"
  in_278/1 -> EPB1/9  "RAW_Byte_5"
  in_279/1 -> EPB1/10  "RAW_Byte_6"
  in_280/1 -> EPB1/11  "RAW_Byte_7"
  in_281/1 -> EPB1/12  "RAW_Byte_8"
  in_282/1 -> HCU3/1  "HybridLimpHome"
  HCU3/1 -> Mux/17  "HCU3"
  in_283/1 -> HCU3/2  "HCU3RollCnt"
  in_284/1 -> HCU3/3  "FuelCutReq"
  in_285/1 -> HCU3/4  "EngCrankType"
  in_286/1 -> HCU3/5  "EngTqIndPermMax_P"
  in_287/1 -> HCU3/6  "EngTqIndPermMax"
  in_288/1 -> HCU3/7  "EngTqBrkReq_P"
  in_289/1 -> HCU3/8  "EngTqBrkReq"
  in_290/1 -> HCU3/9  "EIdleAvail"
  in_291/1 -> HCU3/10  "EIdleActive"
  in_292/1 -> HCU3/11  "EngStpReq"
  in_293/1 -> HCU3/12  "EngStpActive"
  in_294/1 -> HCU3/13  "FuelPumpReq"
  in_295/1 -> HCU3/14  "StarterCrankReq"
  in_296/1 -> HCU3/15  "EngStrtActive"
  in_297/1 -> HCU3/16  "ACDisableReq"
  in_298/1 -> HCU3/17  "RX_Status"
  in_299/1 -> HCU3/18  "RX_Time"
  in_300/1 -> HCU3/19  "RX_DeltaTime"
  in_301/1 -> HCU3/20  "RAW_Byte_1"
  in_302/1 -> HCU3/21  "RAW_Byte_2"
  in_303/1 -> HCU3/22  "RAW_Byte_3"
  in_304/1 -> HCU3/23  "RAW_Byte_4"
  in_305/1 -> HCU3/24  "RAW_Byte_5"
  in_306/1 -> HCU3/25  "RAW_Byte_6"
  in_307/1 -> HCU3/26  "RAW_Byte_7"
  in_308/1 -> HCU3/27  "RAW_Byte_8"
  in_309/1 -> HCU4/1  "STATE_TQI_ETCU_T"
  HCU4/1 -> Mux/18  "HCU4"
  in_310/1 -> HCU4/2  "Start_Stop_STA"
  in_311/1 -> HCU4/3  "Start_Stop_STA_Ind"
  in_312/1 -> HCU4/4  "HEVTransMapReq"
  in_313/1 -> HCU4/5  "MILReq"
  in_314/1 -> HCU4/6  "CAN_TQI_ETCU_GS_T"
  in_315/1 -> HCU4/7  "ISS_Idol_stop_flag"
  in_316/1 -> HCU4/8  "EngIdleSpdSetpt"
  in_317/1 -> HCU4/9  "BSGActTq4EMS_P"
  in_318/1 -> HCU4/10  "BSGActTq4EMS"
  in_319/1 -> HCU4/11  "RX_Status"
  in_320/1 -> HCU4/12  "RX_Time"
  in_321/1 -> HCU4/13  "RX_DeltaTime"
  in_322/1 -> HCU4/14  "RAW_Byte_1"
  in_323/1 -> HCU4/15  "RAW_Byte_2"
  in_324/1 -> HCU4/16  "RAW_Byte_3"
  in_325/1 -> HCU4/17  "RAW_Byte_4"
  in_326/1 -> HCU4/18  "RAW_Byte_5"
  in_327/1 -> HCU4/19  "RAW_Byte_6"
  in_328/1 -> HCU4/20  "RAW_Byte_7"
  in_329/1 -> HCU4/21  "RAW_Byte_8"
  in_330/1 -> HMI1/1  "IGSASwitchMode"
  HMI1/1 -> Mux/19  "HMI1"
  in_331/1 -> HMI1/2  "IGSASet_SpdDec"
  in_332/1 -> HMI1/3  "IGSARes_SpdInc"
  in_333/1 -> HMI1/4  "IGSAOn"
  in_334/1 -> HMI1/5  "LFC_PilotCancel"
  in_335/1 -> HMI1/6  "LFC_PilotOn"
  in_336/1 -> HMI1/7  "FCWWarningMode"
  in_337/1 -> HMI1/8  "LCSEnable"
  in_338/1 -> HMI1/9  "LKAEnable"
  in_339/1 -> HMI1/10  "MAPAEnable"
  in_340/1 -> HMI1/11  "CSCEnable"
  in_341/1 -> HMI1/12  "FCWEnable"
  in_342/1 -> HMI1/13  "AEBEnable"
  in_343/1 -> HMI1/14  "DefMaxACCSetSpeed"
  in_344/1 -> HMI1/15  "ACCSpeedDec"
  in_345/1 -> HMI1/16  "ACCSpeedInc"
  in_346/1 -> HMI1/17  "ACCSet_SpdDec"
  in_347/1 -> HMI1/18  "ACCRes_SpdInc"
  in_348/1 -> HMI1/19  "ACCCancel"
  in_349/1 -> HMI1/20  "ACCOn"
  in_350/1 -> HMI1/21  "ACCTimeGapDec"
  in_351/1 -> HMI1/22  "ACCTimeGapInc"
  in_352/1 -> HMI1/23  "RX_Status"
  in_353/1 -> HMI1/24  "RX_Time"
  in_354/1 -> HMI1/25  "RX_DeltaTime"
  in_355/1 -> HMI1/26  "RAW_Byte_1"
  in_356/1 -> HMI1/27  "RAW_Byte_2"
  in_357/1 -> HMI1/28  "RAW_Byte_3"
  in_358/1 -> HMI1/29  "RAW_Byte_4"
  in_359/1 -> HMI1/30  "RAW_Byte_5"
  in_360/1 -> HMI1/31  "RAW_Byte_6"
  in_361/1 -> HMI1/32  "RAW_Byte_7"
  in_362/1 -> HMI1/33  "RAW_Byte_8"
  in_363/1 -> HMI2/1  "MSAOn_VCU"
  HMI2/1 -> Mux/20  "HMI2"
  in_364/1 -> HMI2/2  "LFCOn_VCU"
  in_365/1 -> HMI2/3  "ACCTimeGapDec_VCU"
  in_366/1 -> HMI2/4  "ACCTimeGapInc_VCU"
  in_367/1 -> HMI2/5  "ACCRes_SpdInc_VCU"
  in_368/1 -> HMI2/6  "ACCSet_SpdDec_VCU"
  in_369/1 -> HMI2/7  "ACCOn_VCU"
  in_370/1 -> HMI2/8  "RX_Status"
  in_371/1 -> HMI2/9  "RX_Time"
  in_372/1 -> HMI2/10  "RX_DeltaTime"
  in_373/1 -> HMI2/11  "RAW_Byte_1"
  in_374/1 -> HMI2/12  "RAW_Byte_2"
  in_375/1 -> HMI2/13  "RAW_Byte_3"
  in_376/1 -> HMI2/14  "RAW_Byte_4"
  in_377/1 -> HMI2/15  "RAW_Byte_5"
  in_378/1 -> HMI2/16  "RAW_Byte_6"
  in_379/1 -> HMI2/17  "RAW_Byte_7"
  in_380/1 -> HMI2/18  "RAW_Byte_8"
  in_381/1 -> Meter1/1  "ODOMETER"
  Meter1/1 -> Mux/21  "Meter1"
  in_382/1 -> Meter1/2  "SeatBelt"
  in_383/1 -> Meter1/3  "LowBrakeFluid_Sta"
  in_384/1 -> Meter1/4  "ParkBrake"
  in_385/1 -> Meter1/5  "RX_Status"
  in_386/1 -> Meter1/6  "RX_Time"
  in_387/1 -> Meter1/7  "RX_DeltaTime"
  in_388/1 -> Meter1/8  "RAW_Byte_1"
  in_389/1 -> Meter1/9  "RAW_Byte_2"
  in_390/1 -> Meter1/10  "RAW_Byte_3"
  in_391/1 -> Meter1/11  "RAW_Byte_4"
  in_392/1 -> Meter1/12  "RAW_Byte_5"
  in_393/1 -> Meter1/13  "RAW_Byte_6"
  in_394/1 -> Meter1/14  "RAW_Byte_7"
  in_395/1 -> Meter1/15  "RAW_Byte_8"
  in_396/1 -> Meter3/1  "Meter_Ind_VehSpeed"
  Meter3/1 -> Mux/22  "Meter3"
  in_397/1 -> Meter3/2  "RX_Status"
  in_398/1 -> Meter3/3  "RX_Time"
  in_399/1 -> Meter3/4  "RX_DeltaTime"
  in_400/1 -> Meter3/5  "RAW_Byte_1"
  in_401/1 -> Meter3/6  "RAW_Byte_2"
  in_402/1 -> Meter3/7  "RAW_Byte_3"
  in_403/1 -> Meter3/8  "RAW_Byte_4"
  in_404/1 -> Meter3/9  "RAW_Byte_5"
  in_405/1 -> Meter3/10  "RAW_Byte_6"
  in_406/1 -> Meter3/11  "RAW_Byte_7"
  in_407/1 -> Meter3/12  "RAW_Byte_8"
  in_408/1 -> NMmADAS/1  "NM_ADAS_SC"
  NMmADAS/1 -> Mux/23  "NMmADAS"
  in_409/1 -> NMmADAS/2  "NM_ADAS_AR"
  in_410/1 -> NMmADAS/3  "NM_ADAS_D_ES"
  in_411/1 -> NMmADAS/4  "NM_ADAS_Zero_Byte"
  in_412/1 -> NMmADAS/5  "RX_Status"
  in_413/1 -> NMmADAS/6  "RX_Time"
  in_414/1 -> NMmADAS/7  "RX_DeltaTime"
  in_415/1 -> NMmADAS/8  "RAW_Byte_1"
  in_416/1 -> NMmADAS/9  "RAW_Byte_2"
  in_417/1 -> NMmADAS/10  "RAW_Byte_3"
  in_418/1 -> NMmADAS/11  "RAW_Byte_4"
  in_419/1 -> NMmADAS/12  "RAW_Byte_5"
  in_420/1 -> NMmADAS/13  "RAW_Byte_6"
  in_421/1 -> NMmADAS/14  "RAW_Byte_7"
  in_422/1 -> NMmADAS/15  "RAW_Byte_8"
  in_423/1 -> SAS1/1  "SAS_CheckSum"
  SAS1/1 -> Mux/24  "SAS1"
  in_424/1 -> SAS1/2  "SAS_MsgCount"
  in_425/1 -> SAS1/3  "SAS_OK"
  in_426/1 -> SAS1/4  "SAS_CAL"
  in_427/1 -> SAS1/5  "SAS_Angle"
  in_428/1 -> SAS1/6  "RX_Status"
  in_429/1 -> SAS1/7  "RX_Time"
  in_430/1 -> SAS1/8  "RX_DeltaTime"
  in_431/1 -> SAS1/9  "RAW_Byte_1"
  in_432/1 -> SAS1/10  "RAW_Byte_2"
  in_433/1 -> SAS1/11  "RAW_Byte_3"
  in_434/1 -> SAS1/12  "RAW_Byte_4"
  in_435/1 -> SAS1/13  "RAW_Byte_5"
  in_436/1 -> SAS1/14  "RAW_Byte_6"
  in_437/1 -> SAS1/15  "RAW_Byte_7"
  in_438/1 -> SAS1/16  "RAW_Byte_8"
  in_439/1 -> TCM1/1  "CAN_N_TM"
  TCM1/1 -> Mux/25  "TCM1"
  in_440/1 -> TCM1/2  "LV_CAN_N_TM_ERR"
  in_441/1 -> TCM1/3  "CAN_GEAR_STATE_NOW"
  in_442/1 -> TCM1/4  "CAN_GEAR_STA_NOW_V"
  in_443/1 -> TCM1/5  "CAN_TQI_ETCU_GS"
  in_444/1 -> TCM1/6  "STATE_CAN_TQI_ETCU"
  in_445/1 -> TCM1/7  "CAN_GEAR_SEL_ETCU"
  in_446/1 -> TCM1/8  "CAN_ETCU_STATE"
  in_447/1 -> TCM1/9  "RX_Status"
  in_448/1 -> TCM1/10  "RX_Time"
  in_449/1 -> TCM1/11  "RX_DeltaTime"
  in_450/1 -> TCM1/12  "RAW_Byte_1"
  in_451/1 -> TCM1/13  "RAW_Byte_2"
  in_452/1 -> TCM1/14  "RAW_Byte_3"
  in_453/1 -> TCM1/15  "RAW_Byte_4"
  in_454/1 -> TCM1/16  "RAW_Byte_5"
  in_455/1 -> TCM1/17  "RAW_Byte_6"
  in_456/1 -> TCM1/18  "RAW_Byte_7"
  in_457/1 -> TCM1/19  "RAW_Byte_8"
  in_458/1 -> TCM2/1  "DR_MODE_IND"
  TCM2/1 -> Mux/26  "TCM2"
  in_459/1 -> TCM2/2  "RX_Status"
  in_460/1 -> TCM2/3  "RX_Time"
  in_461/1 -> TCM2/4  "RX_DeltaTime"
  in_462/1 -> TCM2/5  "RAW_Byte_1"
  in_463/1 -> TCM2/6  "RAW_Byte_2"
  in_464/1 -> TCM2/7  "RAW_Byte_3"
  in_465/1 -> TCM2/8  "RAW_Byte_4"
  in_466/1 -> TCM2/9  "RAW_Byte_5"
  in_467/1 -> TCM2/10  "RAW_Byte_6"
  in_468/1 -> TCM2/11  "RAW_Byte_7"
  in_469/1 -> TCM2/12  "RAW_Byte_8"
  in_470/1 -> VCU1/1  "VCU1_Checksum"
  VCU1/1 -> Mux/27  "VCU1"
  in_471/1 -> VCU1/2  "VCU1_LifeCount"
  in_472/1 -> VCU1/3  "VCUBattVolt"
  in_473/1 -> VCU1/4  "CurVehDec"
  in_474/1 -> VCU1/5  "CurBrakDecReq"
  in_475/1 -> VCU1/6  "CurBrakDecReq_A"
  in_476/1 -> VCU1/7  "CurVehDec_V"
  in_477/1 -> VCU1/8  "DecContMan"
  in_478/1 -> VCU1/9  "ESCBrakStatus"
  in_479/1 -> VCU1/10  "VCUFault"
  in_480/1 -> VCU1/11  "ESCExtBrkAvail"
  in_481/1 -> VCU1/12  "BrakePrefillAvail"
  in_482/1 -> VCU1/13  "DrivBrakSw"
  in_483/1 -> VCU1/14  "EMSTqSrc"
  in_484/1 -> VCU1/15  "EMSExtTqAvail"
  in_485/1 -> VCU1/16  "CurEngTqReq_A"
  in_486/1 -> VCU1/17  "CurEngTqReq"
  in_487/1 -> VCU1/18  "RX_Status"
  in_488/1 -> VCU1/19  "RX_Time"
  in_489/1 -> VCU1/20  "RX_DeltaTime"
  in_490/1 -> VCU1/21  "RAW_Byte_1"
  in_491/1 -> VCU1/22  "RAW_Byte_2"
  in_492/1 -> VCU1/23  "RAW_Byte_3"
  in_493/1 -> VCU1/24  "RAW_Byte_4"
  in_494/1 -> VCU1/25  "RAW_Byte_5"
  in_495/1 -> VCU1/26  "RAW_Byte_6"
  in_496/1 -> VCU1/27  "RAW_Byte_7"
  in_497/1 -> VCU1/28  "RAW_Byte_8"
  in_498/1 -> VCU2/1  "VCU2_Checksum"
  VCU2/1 -> Mux/28  "VCU2"
  in_499/1 -> VCU2/2  "VCU2_LifeCount"
  in_500/1 -> VCU2/3  "CurDriverTqReq"
  in_501/1 -> VCU2/4  "CurDriverTqReq_V"
  in_502/1 -> VCU2/5  "VCU_AccelPedalPosn_V"
  in_503/1 -> VCU2/6  "VCU_AccelPedalPosn"
  in_504/1 -> VCU2/7  "RX_Status"
  in_505/1 -> VCU2/8  "RX_Time"
  in_506/1 -> VCU2/9  "RX_DeltaTime"
  in_507/1 -> VCU2/10  "RAW_Byte_1"
  in_508/1 -> VCU2/11  "RAW_Byte_2"
  in_509/1 -> VCU2/12  "RAW_Byte_3"
  in_510/1 -> VCU2/13  "RAW_Byte_4"
  in_511/1 -> VCU2/14  "RAW_Byte_5"
  in_512/1 -> VCU2/15  "RAW_Byte_6"
  in_513/1 -> VCU2/16  "RAW_Byte_7"
  in_514/1 -> VCU2/17  "RAW_Byte_8"
  Mux/1 -> out/1

== system hcu_main_ADASwEPS/CAN2/ModelClose ==
